simulink model "ee_lithium_pack_cooling"  (R2023a)
settings: Solver=ode23t  StartTime=0.0  StopTime=400  MaxStep=5e-2  RelTol=1e-3  AbsTol=1e-3
PreLoadFcn:
  | ee_lithium_pack_cooling_ini
undefined symbols (not defined in the file): ambient, coolantTemp, Flowrate_vec
libraries: nesl_utility x18, fl_lib x8, ee_battery_module_lib x4
CloseFcn:
  | clear simlog_ee_lithium_pack_cooling
  | 
  | try,close(h1_ssc_lithium_pack_cooling),end
  | clear h1_ssc_lithium_pack_cooling
  | 
  | clear ambient T_vec AH SOC_vec Flowrate_vec
  | clear V0_mat R0_mat R1_mat Tau1_mat R2_mat Tau2_mat
  | clear Ndisc delV0 delR0 delR1 delR2 delAH delLeak
  | clear MdotCp K_cell h_cell
  | clear cell_H cell_W cell_T Ns Np Rext
  | clear coolantQ extHeat AhrVar cellT_ini cellSOC_ini
  | 
  | clear i tout coolantTemp initialPackSOC
  | clear Ns4 Np4 Rext4 coolantQ4
  | clear extHeat4 AhrVar4 cellT_ini4 cellSOC_ini4
Description:
  | Battery Pack Thermal Management
settings Model: Creator=The MathWorks, Inc.  LastModifiedBy=tanis
settings SolverCC: AutoScaleAbsTol=off  ZeroCrossAlgorithm=Adaptive  AlgebraicLoopSolver=TrustRegion  MaxZcPerStep=1
settings DataIOCC: ReturnWorkspaceOutputs=off
settings OptimizationCC: ReuseModelBlockBuffer=off
settings DebuggingCC: IgnoredZcDiagnostic=none  UnconnectedInputMsg=warning  UnconnectedOutputMsg=warning  UnconnectedLineMsg=warning  SymbolicDimsDataTypeCodeGenerationDiagnostic=none
settings ModelReferenceCC: EnableRefExpFcnMdlSchedulingChecks=on
settings SFSimCC: CustomCodeUndefinedFunction=UseInterfaceOnly
settings RTWCC: DLArmComputeVersion=19.05
settings SimscapeCC: SimscapeLogType=all  SimscapeLogSimulationStatistics=on  SimscapeLogName=simlog_ee_lithium_pack_cooling  SimscapeLogDataHistory=250000

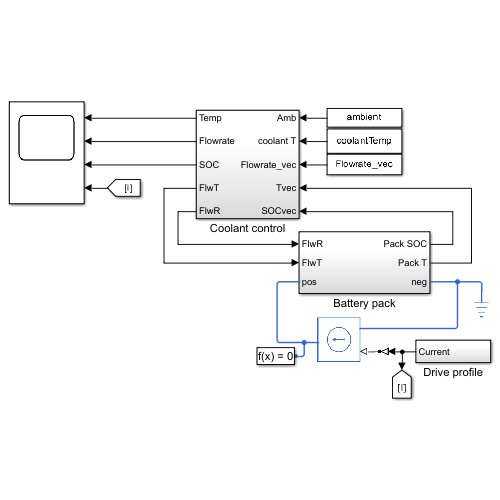
[thumbnail: Simulink's stored preview of the top-level diagram]
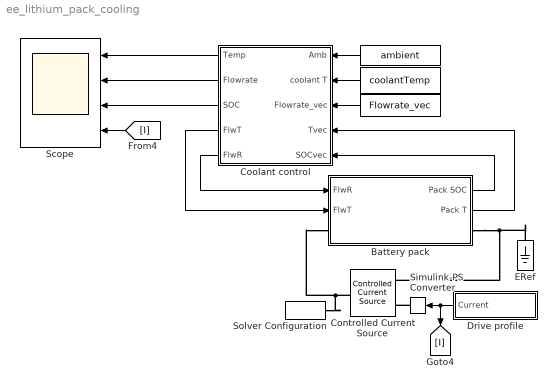
== system ee_lithium_pack_cooling ==
  " " : Constant  Value=coolantTemp
  "    " : Constant  Value=Flowrate_vec
  "       " : Constant  Value=ambient
  Battery pack : Subsystem
  Controlled Current Source : fl_lib/Electrical/Electrical Sources/Controlled Current Source
  Coolant control : Subsystem
  Drive profile : Subsystem
  "ERef " : fl_lib/Electrical/Electrical Elements/Electrical Reference
  Scope : Scope  NumInputPorts=4
  Simulink-PS Converter : nesl_utility/Simulink-PS Converter  PhysicalDomain=network_engine_domain  SubClassName=ps_input  LeftPortType=input  RightPortType=output  PseudoPeriodic=off  Frequencies=[]  NoiseDistribution=none  NoiseParameters=[]  Unit=1  AffineConversion=off  FilteringAndDerivatives=filter  SimscapeFilterOrder=1  InputFilterTimeConstant=0.01  UdotUserProvided=0
  Solver Configuration : nesl_utility/Solver Configuration  PhysicalDomain=network_engine_domain  SubClassName=solver  LeftPortType=input  RightPortType=generic  Tones=[]  Harmonics=[]  SimulateNoise=off  Profile=off  UseLocalSampling=off  EnableSwitchedLinearOptims=on  FrequencyDomain=off  UseCCode=off  RelTol=0.001  AbsTol=1e-06  MinStep=1e-09  ToWorkspace=off  RevertToSquareIcSolve=off  NumHomotopyIterations=100  PhasorMode=off  PhasorModeNumHarmonics=1  ConsistencySolver=NEWTON_FTOL  IndexReductionMethod=DerivativeReplacement  DoDC=off  ResidualTolerance=1e-09  ConsistencyTolSource=GLOBAL  ConsistencyAbsTol=0.001  ConsistencyRelTol=0.001  ConsistencyTolFactor=0.001  UseLocalSolver=off  LocalSolverChoice=NE_BACKWARD_EULER_ADVANCER  ResolveIndetEquations=on  FunctionEvalNumThread=1  LocalSolverSampleTime=0.01  DoFixedCost=off  MaxNonlinIter=3  MaxModeIter=2  ComputeImpulses=off  ImpulseIterations=1  LinearAlgebra=auto  LinearAlgebraNumThread=0  EquationFormulation=NE_TIME_EF  DelaysMemoryBudget=1024  AutomaticFiltering=on  FilteringTimeConstant=0.001  PartitionStorageMethod=AS_NEEDED  PartitionMemoryBudget=1024  PartitionMethod=ROBUST
  wires:
  Coolant control/5(FlwR) -> Battery pack/1(FlwR)
  Coolant control/4(FlwT) -> Battery pack/2(FlwT)
  Drive profile/1(Current) -> [I], Simulink-PS Converter/1
  Battery pack/2(Pack T) -> Coolant control/4(Tvec)
  Battery pack/1(Pack SOC) -> Coolant control/5(SOCvec)
  "    "/1 -> Coolant control/3(Flowrate_vec)
  "       "/1 -> Coolant control/1(Amb)
  " "/1 -> Coolant control/2(coolant T)
  [I] -> Scope/4
  Coolant control/3(SOC) -> Scope/3
  Coolant control/2(Flowrate) -> Scope/2
  Coolant control/1(Temp) -> Scope/1
  connections:
  Simulink-PS Converter/RConn1 -- Controlled Current Source/RConn1
  Controlled Current Source/LConn1 -- Battery pack/LConn1 -- Solver Configuration/RConn1
  Battery pack/RConn1 -- Controlled Current Source/RConn2 -- "ERef "/LConn1

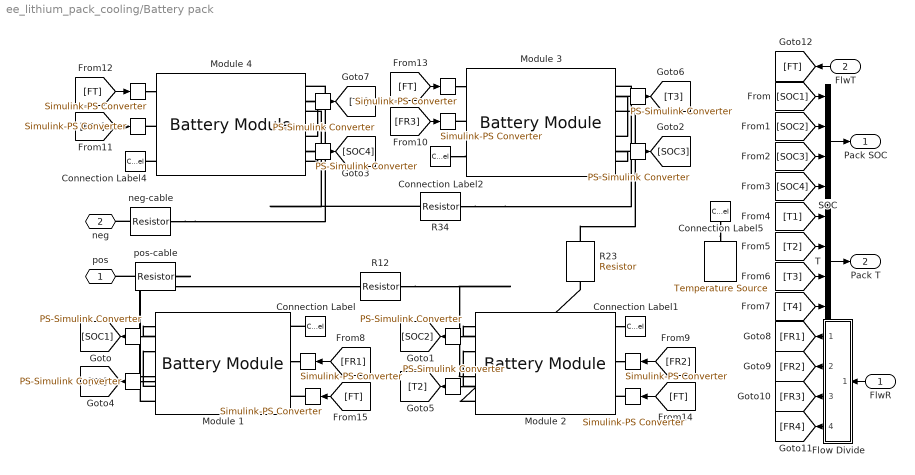
== system ee_lithium_pack_cooling/Battery pack ==
  FlwR : Inport
  FlwT : Inport  Port=2
  " " : nesl_utility/PS-Simulink Converter  PhysicalDomain=network_engine_domain  SubClassName=ps_output  LeftPortType=input  RightPortType=output  PseudoPeriodic=off  Frequencies=[]  VectorFormat=1-D array  Unit=inherit  AffineConversion=off
  "  " : nesl_utility/PS-Simulink Converter  PhysicalDomain=network_engine_domain  SubClassName=ps_output  LeftPortType=input  RightPortType=output  PseudoPeriodic=off  Frequencies=[]  VectorFormat=1-D array  Unit=inherit  AffineConversion=off
  "   " : nesl_utility/PS-Simulink Converter  PhysicalDomain=network_engine_domain  SubClassName=ps_output  LeftPortType=input  RightPortType=output  PseudoPeriodic=off  Frequencies=[]  VectorFormat=1-D array  Unit=inherit  AffineConversion=off
  "    " : nesl_utility/Simulink-PS Converter  PhysicalDomain=network_engine_domain  SubClassName=ps_input  LeftPortType=input  RightPortType=output  PseudoPeriodic=off  Frequencies=[]  NoiseDistribution=none  NoiseParameters=[]  Unit=1  AffineConversion=off  FilteringAndDerivatives=filter  SimscapeFilterOrder=1  InputFilterTimeConstant=0.01  UdotUserProvided=0
  "     " : fl_lib/Thermal/Thermal Sources/Temperature Source  temperature=ambient K
  "      " : nesl_utility/PS-Simulink Converter  PhysicalDomain=network_engine_domain  SubClassName=ps_output  LeftPortType=input  RightPortType=output  PseudoPeriodic=off  Frequencies=[]  VectorFormat=1-D array  Unit=inherit  AffineConversion=off
  "       " : nesl_utility/Simulink-PS Converter  PhysicalDomain=network_engine_domain  SubClassName=ps_input  LeftPortType=input  RightPortType=output  PseudoPeriodic=off  Frequencies=[]  NoiseDistribution=none  NoiseParameters=[]  Unit=1  AffineConversion=off  FilteringAndDerivatives=filter  SimscapeFilterOrder=1  InputFilterTimeConstant=0.01  UdotUserProvided=0
  "         " : nesl_utility/PS-Simulink Converter  PhysicalDomain=network_engine_domain  SubClassName=ps_output  LeftPortType=input  RightPortType=output  PseudoPeriodic=off  Frequencies=[]  VectorFormat=1-D array  Unit=inherit  AffineConversion=off
  "          " : nesl_utility/PS-Simulink Converter  PhysicalDomain=network_engine_domain  SubClassName=ps_output  LeftPortType=input  RightPortType=output  PseudoPeriodic=off  Frequencies=[]  VectorFormat=1-D array  Unit=inherit  AffineConversion=off
  "           " : nesl_utility/Simulink-PS Converter  PhysicalDomain=network_engine_domain  SubClassName=ps_input  LeftPortType=input  RightPortType=output  PseudoPeriodic=off  Frequencies=[]  NoiseDistribution=none  NoiseParameters=[]  Unit=1  AffineConversion=off  FilteringAndDerivatives=filter  SimscapeFilterOrder=1  InputFilterTimeConstant=0.01  UdotUserProvided=0
  "            " : nesl_utility/PS-Simulink Converter  PhysicalDomain=network_engine_domain  SubClassName=ps_output  LeftPortType=input  RightPortType=output  PseudoPeriodic=off  Frequencies=[]  VectorFormat=1-D array  Unit=inherit  AffineConversion=off
  "              " : nesl_utility/Simulink-PS Converter  PhysicalDomain=network_engine_domain  SubClassName=ps_input  LeftPortType=input  RightPortType=output  PseudoPeriodic=off  Frequencies=[]  NoiseDistribution=none  NoiseParameters=[]  Unit=1  AffineConversion=off  FilteringAndDerivatives=filter  SimscapeFilterOrder=1  InputFilterTimeConstant=0.01  UdotUserProvided=0
  "               " : nesl_utility/Simulink-PS Converter  PhysicalDomain=network_engine_domain  SubClassName=ps_input  LeftPortType=input  RightPortType=output  PseudoPeriodic=off  Frequencies=[]  NoiseDistribution=none  NoiseParameters=[]  Unit=1  AffineConversion=off  FilteringAndDerivatives=filter  SimscapeFilterOrder=1  InputFilterTimeConstant=0.01  UdotUserProvided=0
  "                      " : nesl_utility/Simulink-PS Converter  PhysicalDomain=network_engine_domain  SubClassName=ps_input  LeftPortType=input  RightPortType=output  PseudoPeriodic=off  Frequencies=[]  NoiseDistribution=none  NoiseParameters=[]  Unit=1  AffineConversion=off  FilteringAndDerivatives=filter  SimscapeFilterOrder=1  InputFilterTimeConstant=0.01  UdotUserProvided=0
  "                                      " : nesl_utility/PS-Simulink Converter  PhysicalDomain=network_engine_domain  SubClassName=ps_output  LeftPortType=input  RightPortType=output  PseudoPeriodic=off  Frequencies=[]  VectorFormat=1-D array  Unit=inherit  AffineConversion=off
  "                                           " : nesl_utility/Simulink-PS Converter  PhysicalDomain=network_engine_domain  SubClassName=ps_input  LeftPortType=input  RightPortType=output  PseudoPeriodic=off  Frequencies=[]  NoiseDistribution=none  NoiseParameters=[]  Unit=1  AffineConversion=off  FilteringAndDerivatives=filter  SimscapeFilterOrder=1  InputFilterTimeConstant=0.01  UdotUserProvided=0
  "                                                  " : nesl_utility/Simulink-PS Converter  PhysicalDomain=network_engine_domain  SubClassName=ps_input  LeftPortType=input  RightPortType=output  PseudoPeriodic=off  Frequencies=[]  NoiseDistribution=none  NoiseParameters=[]  Unit=1  AffineConversion=off  FilteringAndDerivatives=filter  SimscapeFilterOrder=1  InputFilterTimeConstant=0.01  UdotUserProvided=0
  "                        Flow Divide" : Subsystem
  Connection Label{,1..2,4..5} (5 alike) : ConnectionLabel  Label=Amb
  Module 1 : ee_battery_module_lib/Battery Module  LUTpointsTemp=T_vec K  cellAH=AH A*hr  LUTpointsSOC=SOC_vec  LUTpointsFlowrate=Flowrate_vec kg/s  V0_mat=V0_mat V  prm_dir=simscape.enum.tablebattery.prm_dir.noCurrentDirectionality  R0_mat=R0_mat Ohm  R0_dis_mat=[.03, .015, .002; .04, .017, .008; .039, .012, .006; .027, .013, .021] Ohm  R0_ch_mat=[.03, .015, .002; .04, .017, .008; .039, .012, .006; .027, .013, .021] Ohm  prm_leak=simscape.enum.tablebattery.prm_leak.disabled  Rleak_vec=Rleak Ohm  extrapolation_option=simscape.enum.extrapolation.nearest  prm_dyn=simscape.enum.tablebattery.prm_dyn.rc2  R1_mat=R1_mat Ohm  tau1_mat=Tau1_mat s  R2_mat=R2_mat Ohm  tau2_mat=Tau2_mat s  R3_mat=[.014, .382, .407; .028, .006, .007; .014, .007, .006; .333, .956, .912] Ohm  tau3_mat=[1, 44, 5644; 11, 24, 506; 2, 14, 330; 3310, 13419, 30216] s  R4_mat=[.014, .382, .407; .028, .006, .007; .014, .007, .006; .333, .956, .912] Ohm  tau4_mat=[1, 44, 5644; 11, 24, 506; 2, 14, 330; 3310, 13419, 30216] s  R5_mat=[.014, .382, .407; .028, .006, .007; .014, .007, .006; .333, .956, .912] Ohm  tau5_mat=[1, 44, 5644; 11, 24, 506; 2, 14, 330; 3310, 13419, 30216] s  prm_fade=simscape.enum.tablebattery.prm_fade.equations  N0=Ndisc  dV0=delV0  dR0=delR0  dAH=delAH  dRleak=delLeak  dR1=delR1  dR2=delR2  dR3=0  dR4=0  dR5=0  N0vec=[100, 200, 300]  Tfadevec=[298.15, 323.15] K  dV0vec=[0, 0, 0]  dR0vec=[0, 0, 0]  dAHvec=[0, 0, 0]  dRleakvec=[0, 0, 0]  dR1vec=[0, 0, 0]  dR2vec=[0, 0, 0]  dR3vec=[0, 0, 0]  dR4vec=[0, 0, 0]  dR5vec=[0, 0, 0]  dV0mat=[0, 0; 0, 0; 0, 0]  dR0mat=[0, 0; 0, 0; 0, 0]  dAHmat=[0, 0; 0, 0; 0, 0]  dRleakmat=[0, 0; 0, 0; 0, 0]  dR1mat=[0, 0; 0, 0; 0, 0]  dR2mat=[0, 0; 0, 0; 0, 0]  dR3mat=[0, 0; 0, 0; 0, 0]  dR4mat=[0, 0; 0, 0; 0, 0]  dR5mat=[0, 0; 0, 0; 0, 0]  cellThermalMass=MdotCp J/K  cellThermalCond=K_cell W/(m*K)  cellHeatTrCoeff=h_cell W/(m^2*K)  Ns=Ns  Np=Np  cellTypeSelection=ee_battery_module.batteryTypeSelection.Pouch  cellHeight=cell_H m  cellWidth=cell_W m  cellThickness=cell_T m  cellDiameter=0.018 m  cellCylinLine=3  moduleExternalR=Rext Ohm  moduleCellBalancing=ee_battery_module.batteryCellBalancing.None  passiveShuntR=shuntR Ohm  passiveSWclosedR=swClosedR Ohm  passiveSWopenCond=swOpenC 1/Ohm  passiveSWthreshold=swThreshold  moduleCooling=coolantQ W/K  moduleExtHeat=extHeat W  cellTemp=cellT_ini K  cellSOC=cellSOC_ini  moduleCellAHpercentVar=AhrVar  moduleCellLeakPercentVar=RleakVar
      settings: InternalSimscapePortConfiguration="{\"Bottom\":[],\"Left\":[{\"id\":\"outputCellSOC\",\"label\":\"SOC\",\"type\":\"output\"},{\"id\":\"outputCellTemp\",\"label\":\"Temp\",\"type\":\"output\"}],\"Right\":[{\"id\":\"H\",\"label\":\"Amb\",\"type\":\"foundation.thermal.thermal\"},{\"id\":\"frac\",\"label\":\"FlwR\",\"type\":\"input\"},{\"id\":\"delT\",\"label\":\"FlwT\",\"type\":\"input\"}],\"Top\":[{\"id\":\"p\",\"label\":\"pos\",\"type\":\"foundation.electrical.electrical\"},{\"id\":\"n\",\"label\":\"neg\",\"type\":\"foundation.electrical.electrical\"}]}"
  Module 2 : ee_battery_module_lib/Battery Module  LUTpointsTemp=T_vec K  cellAH=AH A*hr  LUTpointsSOC=SOC_vec  LUTpointsFlowrate=Flowrate_vec kg/s  V0_mat=V0_mat V  prm_dir=simscape.enum.tablebattery.prm_dir.noCurrentDirectionality  R0_mat=R0_mat Ohm  R0_dis_mat=[.03, .015, .002; .04, .017, .008; .039, .012, .006; .027, .013, .021] Ohm  R0_ch_mat=[.03, .015, .002; .04, .017, .008; .039, .012, .006; .027, .013, .021] Ohm  prm_leak=simscape.enum.tablebattery.prm_leak.disabled  Rleak_vec=Rleak Ohm  extrapolation_option=simscape.enum.extrapolation.nearest  prm_dyn=simscape.enum.tablebattery.prm_dyn.rc2  R1_mat=R1_mat Ohm  tau1_mat=Tau1_mat s  R2_mat=R2_mat Ohm  tau2_mat=Tau2_mat s  R3_mat=[.014, .382, .407; .028, .006, .007; .014, .007, .006; .333, .956, .912] Ohm  tau3_mat=[1, 44, 5644; 11, 24, 506; 2, 14, 330; 3310, 13419, 30216] s  R4_mat=[.014, .382, .407; .028, .006, .007; .014, .007, .006; .333, .956, .912] Ohm  tau4_mat=[1, 44, 5644; 11, 24, 506; 2, 14, 330; 3310, 13419, 30216] s  R5_mat=[.014, .382, .407; .028, .006, .007; .014, .007, .006; .333, .956, .912] Ohm  tau5_mat=[1, 44, 5644; 11, 24, 506; 2, 14, 330; 3310, 13419, 30216] s  prm_fade=simscape.enum.tablebattery.prm_fade.equations  N0=Ndisc  dV0=delV0  dR0=delR0  dAH=delAH  dRleak=delLeak  dR1=delR1  dR2=delR2  dR3=0  dR4=0  dR5=0  N0vec=[100, 200, 300]  Tfadevec=[298.15, 323.15] K  dV0vec=[0, 0, 0]  dR0vec=[0, 0, 0]  dAHvec=[0, 0, 0]  dRleakvec=[0, 0, 0]  dR1vec=[0, 0, 0]  dR2vec=[0, 0, 0]  dR3vec=[0, 0, 0]  dR4vec=[0, 0, 0]  dR5vec=[0, 0, 0]  dV0mat=[0, 0; 0, 0; 0, 0]  dR0mat=[0, 0; 0, 0; 0, 0]  dAHmat=[0, 0; 0, 0; 0, 0]  dRleakmat=[0, 0; 0, 0; 0, 0]  dR1mat=[0, 0; 0, 0; 0, 0]  dR2mat=[0, 0; 0, 0; 0, 0]  dR3mat=[0, 0; 0, 0; 0, 0]  dR4mat=[0, 0; 0, 0; 0, 0]  dR5mat=[0, 0; 0, 0; 0, 0]  cellThermalMass=MdotCp J/K  cellThermalCond=K_cell W/(m*K)  cellHeatTrCoeff=h_cell W/(m^2*K)  Ns=Ns  Np=Np  cellTypeSelection=ee_battery_module.batteryTypeSelection.Pouch  cellHeight=cell_H m  cellWidth=cell_W m  cellThickness=cell_T m  cellDiameter=0.018 m  cellCylinLine=3  moduleExternalR=Rext Ohm  moduleCellBalancing=ee_battery_module.batteryCellBalancing.None  passiveShuntR=shuntR Ohm  passiveSWclosedR=swClosedR Ohm  passiveSWopenCond=swOpenC 1/Ohm  passiveSWthreshold=swThreshold  moduleCooling=coolantQ W/K  moduleExtHeat=extHeat W  cellTemp=cellT_ini K  cellSOC=cellSOC_ini  moduleCellAHpercentVar=AhrVar  moduleCellLeakPercentVar=RleakVar
      settings: InternalSimscapePortConfiguration="{\"Bottom\":[],\"Left\":[{\"id\":\"outputCellSOC\",\"label\":\"SOC\",\"type\":\"output\"},{\"id\":\"outputCellTemp\",\"label\":\"Temp\",\"type\":\"output\"}],\"Right\":[{\"id\":\"H\",\"label\":\"Amb\",\"type\":\"foundation.thermal.thermal\"},{\"id\":\"frac\",\"label\":\"FlwR\",\"type\":\"input\"},{\"id\":\"delT\",\"label\":\"FlwT\",\"type\":\"input\"}],\"Top\":[{\"id\":\"p\",\"label\":\"pos\",\"type\":\"foundation.electrical.electrical\"},{\"id\":\"n\",\"label\":\"neg\",\"type\":\"foundation.electrical.electrical\"}]}"
  Module 3 : ee_battery_module_lib/Battery Module  LUTpointsTemp=T_vec K  cellAH=AH A*hr  LUTpointsSOC=SOC_vec  LUTpointsFlowrate=Flowrate_vec kg/s  V0_mat=V0_mat V  prm_dir=simscape.enum.tablebattery.prm_dir.noCurrentDirectionality  R0_mat=R0_mat Ohm  R0_dis_mat=[.03, .015, .002; .04, .017, .008; .039, .012, .006; .027, .013, .021] Ohm  R0_ch_mat=[.03, .015, .002; .04, .017, .008; .039, .012, .006; .027, .013, .021] Ohm  prm_leak=simscape.enum.tablebattery.prm_leak.disabled  Rleak_vec=Rleak Ohm  extrapolation_option=simscape.enum.extrapolation.nearest  prm_dyn=simscape.enum.tablebattery.prm_dyn.rc2  R1_mat=R1_mat Ohm  tau1_mat=Tau1_mat s  R2_mat=R2_mat Ohm  tau2_mat=Tau2_mat s  R3_mat=[.014, .382, .407; .028, .006, .007; .014, .007, .006; .333, .956, .912] Ohm  tau3_mat=[1, 44, 5644; 11, 24, 506; 2, 14, 330; 3310, 13419, 30216] s  R4_mat=[.014, .382, .407; .028, .006, .007; .014, .007, .006; .333, .956, .912] Ohm  tau4_mat=[1, 44, 5644; 11, 24, 506; 2, 14, 330; 3310, 13419, 30216] s  R5_mat=[.014, .382, .407; .028, .006, .007; .014, .007, .006; .333, .956, .912] Ohm  tau5_mat=[1, 44, 5644; 11, 24, 506; 2, 14, 330; 3310, 13419, 30216] s  prm_fade=simscape.enum.tablebattery.prm_fade.equations  N0=Ndisc  dV0=delV0  dR0=delR0  dAH=delAH  dRleak=delLeak  dR1=delR1  dR2=delR2  dR3=0  dR4=0  dR5=0  N0vec=[100, 200, 300]  Tfadevec=[298.15, 323.15] K  dV0vec=[0, 0, 0]  dR0vec=[0, 0, 0]  dAHvec=[0, 0, 0]  dRleakvec=[0, 0, 0]  dR1vec=[0, 0, 0]  dR2vec=[0, 0, 0]  dR3vec=[0, 0, 0]  dR4vec=[0, 0, 0]  dR5vec=[0, 0, 0]  dV0mat=[0, 0; 0, 0; 0, 0]  dR0mat=[0, 0; 0, 0; 0, 0]  dAHmat=[0, 0; 0, 0; 0, 0]  dRleakmat=[0, 0; 0, 0; 0, 0]  dR1mat=[0, 0; 0, 0; 0, 0]  dR2mat=[0, 0; 0, 0; 0, 0]  dR3mat=[0, 0; 0, 0; 0, 0]  dR4mat=[0, 0; 0, 0; 0, 0]  dR5mat=[0, 0; 0, 0; 0, 0]  cellThermalMass=MdotCp J/K  cellThermalCond=K_cell W/(m*K)  cellHeatTrCoeff=h_cell W/(m^2*K)  Ns=Ns  Np=Np  cellTypeSelection=ee_battery_module.batteryTypeSelection.Pouch  cellHeight=cell_H m  cellWidth=cell_W m  cellThickness=cell_T m  cellDiameter=0.018 m  cellCylinLine=3  moduleExternalR=Rext Ohm  moduleCellBalancing=ee_battery_module.batteryCellBalancing.None  passiveShuntR=shuntR Ohm  passiveSWclosedR=swClosedR Ohm  passiveSWopenCond=swOpenC 1/Ohm  passiveSWthreshold=swThreshold  moduleCooling=coolantQ W/K  moduleExtHeat=extHeat W  cellTemp=cellT_ini K  cellSOC=cellSOC_ini  moduleCellAHpercentVar=AhrVar  moduleCellLeakPercentVar=RleakVar
      settings: InternalSimscapePortConfiguration="{\"Bottom\":[],\"Left\":[{\"id\":\"outputCellSOC\",\"label\":\"SOC\",\"type\":\"output\"},{\"id\":\"outputCellTemp\",\"label\":\"Temp\",\"type\":\"output\"}],\"Right\":[{\"id\":\"H\",\"label\":\"Amb\",\"type\":\"foundation.thermal.thermal\"},{\"id\":\"frac\",\"label\":\"FlwR\",\"type\":\"input\"},{\"id\":\"delT\",\"label\":\"FlwT\",\"type\":\"input\"}],\"Top\":[{\"id\":\"p\",\"label\":\"pos\",\"type\":\"foundation.electrical.electrical\"},{\"id\":\"n\",\"label\":\"neg\",\"type\":\"foundation.electrical.electrical\"}]}"
  Module 4 : ee_battery_module_lib/Battery Module  LUTpointsTemp=T_vec K  cellAH=AH A*hr  LUTpointsSOC=SOC_vec  LUTpointsFlowrate=Flowrate_vec kg/s  V0_mat=V0_mat V  prm_dir=simscape.enum.tablebattery.prm_dir.noCurrentDirectionality  R0_mat=R0_mat Ohm  R0_dis_mat=[.03, .015, .002; .04, .017, .008; .039, .012, .006; .027, .013, .021] Ohm  R0_ch_mat=[.03, .015, .002; .04, .017, .008; .039, .012, .006; .027, .013, .021] Ohm  prm_leak=simscape.enum.tablebattery.prm_leak.disabled  Rleak_vec=Rleak Ohm  extrapolation_option=simscape.enum.extrapolation.nearest  prm_dyn=simscape.enum.tablebattery.prm_dyn.rc2  R1_mat=R1_mat Ohm  tau1_mat=Tau1_mat s  R2_mat=R2_mat Ohm  tau2_mat=Tau2_mat s  R3_mat=[.014, .382, .407; .028, .006, .007; .014, .007, .006; .333, .956, .912] Ohm  tau3_mat=[1, 44, 5644; 11, 24, 506; 2, 14, 330; 3310, 13419, 30216] s  R4_mat=[.014, .382, .407; .028, .006, .007; .014, .007, .006; .333, .956, .912] Ohm  tau4_mat=[1, 44, 5644; 11, 24, 506; 2, 14, 330; 3310, 13419, 30216] s  R5_mat=[.014, .382, .407; .028, .006, .007; .014, .007, .006; .333, .956, .912] Ohm  tau5_mat=[1, 44, 5644; 11, 24, 506; 2, 14, 330; 3310, 13419, 30216] s  prm_fade=simscape.enum.tablebattery.prm_fade.equations  N0=Ndisc  dV0=delV0  dR0=delR0  dAH=delAH  dRleak=delLeak  dR1=delR1  dR2=delR2  dR3=0  dR4=0  dR5=0  N0vec=[100, 200, 300]  Tfadevec=[298.15, 323.15] K  dV0vec=[0, 0, 0]  dR0vec=[0, 0, 0]  dAHvec=[0, 0, 0]  dRleakvec=[0, 0, 0]  dR1vec=[0, 0, 0]  dR2vec=[0, 0, 0]  dR3vec=[0, 0, 0]  dR4vec=[0, 0, 0]  dR5vec=[0, 0, 0]  dV0mat=[0, 0; 0, 0; 0, 0]  dR0mat=[0, 0; 0, 0; 0, 0]  dAHmat=[0, 0; 0, 0; 0, 0]  dRleakmat=[0, 0; 0, 0; 0, 0]  dR1mat=[0, 0; 0, 0; 0, 0]  dR2mat=[0, 0; 0, 0; 0, 0]  dR3mat=[0, 0; 0, 0; 0, 0]  dR4mat=[0, 0; 0, 0; 0, 0]  dR5mat=[0, 0; 0, 0; 0, 0]  cellThermalMass=MdotCp J/K  cellThermalCond=K_cell W/(m*K)  cellHeatTrCoeff=h_cell W/(m^2*K)  Ns=Ns4  Np=Np4  cellTypeSelection=ee_battery_module.batteryTypeSelection.Pouch  cellHeight=cell_H m  cellWidth=cell_W m  cellThickness=cell_T m  cellDiameter=0.018 m  cellCylinLine=3  moduleExternalR=Rext4 Ohm  moduleCellBalancing=ee_battery_module.batteryCellBalancing.None  passiveShuntR=shuntR Ohm  passiveSWclosedR=swClosedR Ohm  passiveSWopenCond=swOpenC 1/Ohm  passiveSWthreshold=swThreshold  moduleCooling=coolantQ4 W/K  moduleExtHeat=extHeat4 W  cellTemp=cellT_ini4 K  cellSOC=cellSOC_ini4  moduleCellAHpercentVar=AhrVar4  moduleCellLeakPercentVar=RleakVar
      settings: InternalSimscapePortConfiguration="{\"Bottom\":[],\"Left\":[{\"id\":\"outputCellSOC\",\"label\":\"SOC\",\"type\":\"output\"},{\"id\":\"outputCellTemp\",\"label\":\"Temp\",\"type\":\"output\"}],\"Right\":[{\"id\":\"H\",\"label\":\"Amb\",\"type\":\"foundation.thermal.thermal\"},{\"id\":\"frac\",\"label\":\"FlwR\",\"type\":\"input\"},{\"id\":\"delT\",\"label\":\"FlwT\",\"type\":\"input\"}],\"Top\":[{\"id\":\"p\",\"label\":\"pos\",\"type\":\"foundation.electrical.electrical\"},{\"id\":\"n\",\"label\":\"neg\",\"type\":\"foundation.electrical.electrical\"}]}"
  R12 : fl_lib/Electrical/Electrical Elements/Resistor  R=0.001 Ohm  i_specify=off  i_priority=None  i=0 A  i_nominal_specify=off  i_nominal_unit=A  i_nominal_value=1  v_specify=off  v_priority=None  v=0 V  v_nominal_specify=off  v_nominal_unit=V  v_nominal_value=1
  R23 : fl_lib/Electrical/Electrical Elements/Resistor  R=0.001 Ohm  i_specify=off  i_priority=None  i=0 A  i_nominal_specify=off  i_nominal_unit=A  i_nominal_value=1  v_specify=off  v_priority=None  v=0 V  v_nominal_specify=off  v_nominal_unit=V  v_nominal_value=1
  R34 : fl_lib/Electrical/Electrical Elements/Resistor  R=0.001 Ohm  i_specify=off  i_priority=None  i=0 A  i_nominal_specify=off  i_nominal_unit=A  i_nominal_value=1  v_specify=off  v_priority=None  v=0 V  v_nominal_specify=off  v_nominal_unit=V  v_nominal_value=1
  SOC : Concatenate  NumInputs=4
  T : Concatenate  NumInputs=4
  neg-cable : fl_lib/Electrical/Electrical Elements/Resistor  R=0.001 Ohm  i_specify=off  i_priority=None  i=0 A  i_nominal_specify=off  i_nominal_unit=A  i_nominal_value=1  v_specify=off  v_priority=None  v=0 V  v_nominal_specify=off  v_nominal_unit=V  v_nominal_value=1
  pos-cable : fl_lib/Electrical/Electrical Elements/Resistor  R=0.001 Ohm  i_specify=off  i_priority=None  i=0 A  i_nominal_specify=off  i_nominal_unit=A  i_nominal_value=1  v_specify=off  v_priority=None  v=0 V  v_nominal_specify=off  v_nominal_unit=V  v_nominal_value=1
  pos : PMIOPort  Side=Left
  neg : PMIOPort  Port=2  Side=Right
  Pack SOC : Outport
  Pack T : Outport  Port=2
  wires:
  "  "/1 -> [SOC1]
  "      "/1 -> [SOC2]
  "          "/1 -> [SOC3]
  "            "/1 -> [SOC4]
  [SOC1] -> SOC/1
  [SOC2] -> SOC/2
  [SOC3] -> SOC/3
  [SOC4] -> SOC/4
  [T3] -> T/3
  [T4] -> T/4
  [T2] -> T/2
  [T1] -> T/1
  " "/1 -> [T1]
  "   "/1 -> [T2]
  "         "/1 -> [T3]
  "                                      "/1 -> [T4]
  [FR1] -> "    "/1
  [FR2] -> "       "/1
  [FR3] -> "                      "/1
  [FR4] -> "           "/1
  [FT] -> "               "/1
  [FT] -> "              "/1
  [FT] -> "                                                  "/1
  [FT] -> "                                           "/1
  FlwT/1 -> [FT]
  SOC/1 -> Pack SOC/1
  T/1 -> Pack T/1
  FlwR/1 -> "                        Flow Divide"/1(In1)
  "                        Flow Divide"/1(Out1) -> [FR1]
  "                        Flow Divide"/2(Out2) -> [FR2]
  "                        Flow Divide"/3(Out3) -> [FR3]
  "                        Flow Divide"/4(Out4) -> [FR4]
  connections:
  "              "/RConn1 -- Module 3/RConn3
  Module 4/RConn2 -- "           "/RConn1
  " "/LConn1 -- Module 1/LConn2
  "            "/LConn1 -- Module 4/LConn1
  "      "/LConn1 -- Module 2/LConn1
  "                                      "/LConn1 -- Module 4/LConn2
  "   "/LConn1 -- Module 2/LConn2
  "               "/RConn1 -- Module 4/RConn3
  Module 3/RConn2 -- "                      "/RConn1
  Module 2/RConn2 -- "       "/RConn1
  "  "/LConn1 -- Module 1/LConn1
  "          "/LConn1 -- Module 3/LConn1
  "         "/LConn1 -- Module 3/LConn2
  Connection Label/LConn1 -- Module 1/RConn1
  Module 2/RConn1 -- Connection Label1/LConn1
  Connection Label2/LConn1 -- Module 3/RConn1
  Module 4/RConn1 -- Connection Label4/LConn1
  Connection Label5/LConn1 -- "     "/LConn1
  Module 1/RConn2 -- "    "/RConn1
  "                                                  "/RConn1 -- Module 2/RConn3
  "                                           "/RConn1 -- Module 1/RConn3
  Module 1/LConn4 -- R12/LConn1
  R12/RConn1 -- Module 2/LConn3
  R34/LConn1 -- Module 3/LConn4
  R34/RConn1 -- Module 4/LConn3
  R23/RConn1 -- Module 3/LConn3
  Module 2/LConn4 -- R23/LConn1
  neg-cable/RConn1 -- neg/RConn1
  neg-cable/LConn1 -- Module 4/LConn4
  pos-cable/LConn1 -- pos/RConn1
  pos-cable/RConn1 -- Module 1/LConn3

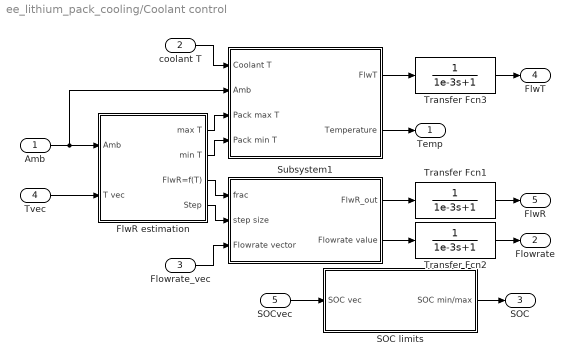
== system ee_lithium_pack_cooling/Coolant control ==
  Amb : Inport
  coolant T : Inport  Port=2
  Flowrate_vec : Inport  Port=3
  Tvec : Inport  Port=4
  SOCvec : Inport  Port=5
  "   " : Subsystem
  FlwR estimation : Subsystem
  SOC limits : Subsystem
  Subsystem1 : Subsystem
  Transfer Fcn1 : TransferFcn  Denominator=[1e-3 1]
  Transfer Fcn2 : TransferFcn  Denominator=[1e-3 1]
  Transfer Fcn3 : TransferFcn  Denominator=[1e-3 1]
  Temp : Outport
  Flowrate : Outport  Port=2
  SOC : Outport  Port=3
  FlwT : Outport  Port=4
  FlwR : Outport  Port=5
  wires:
  Transfer Fcn1/1 -> FlwR/1
  Transfer Fcn2/1 -> Flowrate/1
  Transfer Fcn3/1 -> FlwT/1
  SOCvec/1 -> SOC limits/1(SOC vec)
  SOC limits/1(SOC min/max) -> SOC/1
  Tvec/1 -> FlwR estimation/2(T vec)
  coolant T/1 -> "   "/1(Coolant T)
  FlwR estimation/1(max T) -> "   "/3(Pack max T)
  FlwR estimation/2(min T) -> "   "/4(Pack min T)
  "   "/1(FlwT) -> Transfer Fcn3/1
  "   "/2(Temperature) -> Temp/1
  FlwR estimation/3(FlwR=f(T)) -> Subsystem1/1(frac)
  FlwR estimation/4(Step) -> Subsystem1/2(step size)
  Subsystem1/1(FlwR_out) -> Transfer Fcn1/1
  Subsystem1/2(Flowrate value) -> Transfer Fcn2/1
  Flowrate_vec/1 -> Subsystem1/3(Flowrate vector)
  Amb/1 -> FlwR estimation/1(Amb), "   "/2(Amb)

== system ee_lithium_pack_cooling/Drive profile ==
  Constant3 : Constant  Value=-1
  From File : FromFile  FileName=ee_lithium_pack_cooling_Ivst.mat  SampleTime=0
  Product : Product
  Current : Outport
  wires:
  Product/1 -> Current/1
  From File/1 -> Product/1
  Constant3/1 -> Product/2

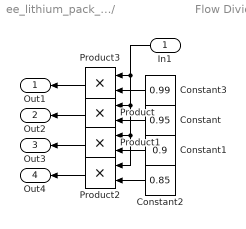
== system ee_lithium_pack_cooling/Battery pack/                        Flow Divide ==
  In1 : Inport
  Constant : Constant  Value=0.95
  Constant1 : Constant  Value=0.9
  Constant2 : Constant  Value=0.85
  Constant3 : Constant  Value=0.99
  Product{,1..3} (4 alike) : Product
  Out1 : Outport
  Out2 : Outport  Port=2
  Out3 : Outport  Port=3
  Out4 : Outport  Port=4
  wires:
  Constant1/1 -> Product1/2
  Constant/1 -> Product/2
  Product/1 -> Out2/1
  In1/1 -> Product2/1, Product1/1, Product/1, Product3/1
  Constant3/1 -> Product3/2
  Product1/1 -> Out3/1
  Constant2/1 -> Product2/2
  Product3/1 -> Out1/1
  Product2/1 -> Out4/1

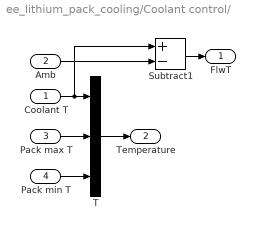
== system ee_lithium_pack_cooling/Coolant control/    ==
  Coolant T : Inport
  Amb : Inport  Port=2
  Pack max T : Inport  Port=3
  Pack min T : Inport  Port=4
  Subtract1 : Sum  Inputs=+-
  T : Concatenate  NumInputs=3
  FlwT : Outport
  Temperature : Outport  Port=2
  wires:
  T/1 -> Temperature/1
  Pack min T/1 -> T/3
  Subtract1/1 -> FlwT/1
  Pack max T/1 -> T/2
  Coolant T/1 -> Subtract1/1, T/1
  Amb/1 -> Subtract1/2

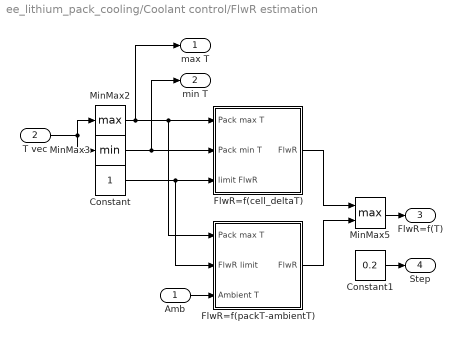
== system ee_lithium_pack_cooling/Coolant control/FlwR estimation ==
  Amb : Inport
  T vec : Inport  Port=2
  Constant : Constant
  Constant1 : Constant  Value=0.2
  FlwR=f(cell_deltaT) : Subsystem
  FlwR=f(packT-ambientT) : Subsystem
  MinMax2 : MinMax  Function=max  ZeroCross=off
  MinMax3 : MinMax  ZeroCross=off
  MinMax5 : MinMax  Function=max  Inputs=2  ZeroCross=off
  max T : Outport
  min T : Outport  Port=2
  FlwR=f(T) : Outport  Port=3
  Step : Outport  Port=4
  wires:
  Constant/1 -> FlwR=f(packT-ambientT)/2(FlwR limit), FlwR=f(cell_deltaT)/3(limit FlwR)
  Constant1/1 -> Step/1
  MinMax3/1 -> min T/1, FlwR=f(cell_deltaT)/2(Pack min T)
  MinMax2/1 -> FlwR=f(packT-ambientT)/1(Pack max T), FlwR=f(cell_deltaT)/1(Pack max T), max T/1
  T vec/1 -> MinMax3/1, MinMax2/1
  MinMax5/1 -> FlwR=f(T)/1
  FlwR=f(cell_deltaT)/1(FlwR) -> MinMax5/1
  Amb/1 -> FlwR=f(packT-ambientT)/3(Ambient T)
  FlwR=f(packT-ambientT)/1(FlwR) -> MinMax5/2

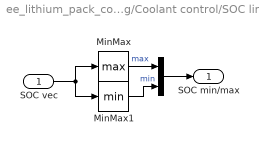
== system ee_lithium_pack_cooling/Coolant control/SOC limits ==
  SOC vec : Inport
  " " : Concatenate
  MinMax : MinMax  Function=max  ZeroCross=off
  MinMax1 : MinMax  ZeroCross=off
  SOC min/max : Outport
  wires:
  MinMax1/1 -> " "/2  "min"
  SOC vec/1 -> MinMax1/1, MinMax/1
  " "/1 -> SOC min/max/1
  MinMax/1 -> " "/1  "max"

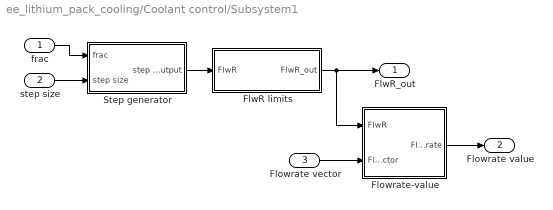
== system ee_lithium_pack_cooling/Coolant control/Subsystem1 ==
  frac : Inport
  step size : Inport  Port=2
  Flowrate vector : Inport  Port=3
  Flowrate-value : Subsystem
  FlwR limits : Subsystem
  Step generator : Subsystem
  FlwR_out : Outport
  Flowrate value : Outport  Port=2
  wires:
  step size/1 -> Step generator/2(step size)
  Flowrate-value/1(Flowrate) -> Flowrate value/1
  Flowrate vector/1 -> Flowrate-value/2(Flowrate vector)
  Step generator/1(step output) -> FlwR limits/1(FlwR)
  frac/1 -> Step generator/1(frac)
  FlwR limits/1(FlwR_out) -> FlwR_out/1, Flowrate-value/1(FlwR)

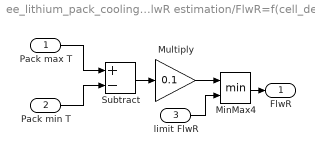
== system ee_lithium_pack_cooling/Coolant control/FlwR estimation/FlwR=f(cell_deltaT) ==
  Pack max T : Inport
  Pack min T : Inport  Port=2
  limit FlwR : Inport  Port=3
  MinMax4 : MinMax  Inputs=2  ZeroCross=off
  Multiply : Gain  Gain=0.1
  Subtract : Sum  Inputs=+-
  FlwR : Outport
  wires:
  Subtract/1 -> Multiply/1
  limit FlwR/1 -> MinMax4/2
  Multiply/1 -> MinMax4/1
  Pack max T/1 -> Subtract/1
  MinMax4/1 -> FlwR/1
  Pack min T/1 -> Subtract/2

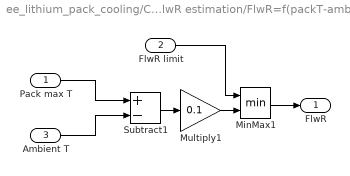
== system ee_lithium_pack_cooling/Coolant control/FlwR estimation/FlwR=f(packT-ambientT) ==
  Pack max T : Inport
  FlwR limit : Inport  Port=2
  Ambient T : Inport  Port=3
  MinMax1 : MinMax  Inputs=2  ZeroCross=off
  Multiply1 : Gain  Gain=0.1
  Subtract1 : Sum  Inputs=+-
  FlwR : Outport
  wires:
  Subtract1/1 -> Multiply1/1
  Multiply1/1 -> MinMax1/2
  FlwR limit/1 -> MinMax1/1
  Pack max T/1 -> Subtract1/1
  MinMax1/1 -> FlwR/1
  Ambient T/1 -> Subtract1/2

== system ee_lithium_pack_cooling/Coolant control/Subsystem1/Flowrate-value ==
  FlwR : Inport
  Flowrate vector : Inport  Port=2
  MinMax6 : MinMax  Function=max  ZeroCross=off
  Product : Product
  Flowrate : Outport
  wires:
  MinMax6/1 -> Product/2
  FlwR/1 -> Product/1
  Product/1 -> Flowrate/1
  Flowrate vector/1 -> MinMax6/1

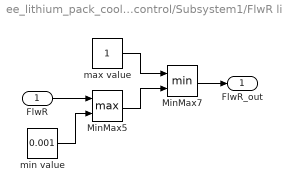
== system ee_lithium_pack_cooling/Coolant control/Subsystem1/FlwR limits ==
  FlwR : Inport
  MinMax5 : MinMax  Function=max  Inputs=2  ZeroCross=off
  MinMax7 : MinMax  Inputs=2  ZeroCross=off
  max value : Constant
  min value : Constant  Value=0.001
  FlwR_out : Outport
  wires:
  min value/1 -> MinMax5/2
  max value/1 -> MinMax7/1
  FlwR/1 -> MinMax5/1
  MinMax5/1 -> MinMax7/2
  MinMax7/1 -> FlwR_out/1

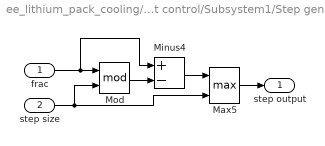
== system ee_lithium_pack_cooling/Coolant control/Subsystem1/Step generator ==
  frac : Inport
  step size : Inport  Port=2
  Max5 : MinMax  Function=max  Inputs=2  ZeroCross=off
  Minus4 : Sum  Inputs=+-
  Mod : Math  Operator=mod
  step output : Outport
  wires:
  Minus4/1 -> Max5/1
  Mod/1 -> Minus4/2
  step size/1 -> Max5/2, Mod/2
  Max5/1 -> step output/1
  frac/1 -> Minus4/1, Mod/1
